simulink model "PID_Tuning"  (R2018a)
settings: Solver=ode45  StartTime=0.0  StopTime=30  RelTol=1e-3  EnableMultiTasking=on
PostLoadFcn:
  | plot_timeseries(Simulation_results);
undefined symbols (not defined in the file or in its folder): A, B, C, D, h, sigbuilder_block
libraries: simulink x4
settings Model: Creator=rbabuska  LastModifiedBy=TU Delf SID
settings DataIOCC: LimitDataPoints=on  SaveFormat=Array
settings OptimizationCC: ExpressionDepthLimit=2147483647  LifeSpan=inf
settings DebuggingCC: AllowSymbolicDim=off  StateNameClashWarn=warning  SFUnexpectedBacktrackingDiag=warning  SFNoUnconditionalDefaultTransitionDiag=warning  SFExecutionAtInitializationDiag=none
settings HardwareCC: ProdBitPerPointer=32  ProdBitPerSizeT=32  ProdBitPerPtrDiffT=32  ProdLargestAtomicFloat=None  ProdIntDivRoundTo=Undefined  ProdEndianess=Unspecified  ProdWordSize=32  ProdHWDeviceType=32-bit Generic
settings ModelReferenceCC: PropagateSignalLabelsOutOfModel=off
settings CodeAppCC: StateflowObjectComments=on
settings GRTTargetCC: TargetLangStandard=C89/C90 (ANSI)  GeneratePreprocessorConditionals=Disable all  CombineOutputUpdateFcns=off  GRTInterface=on
settings ConfigComp: CovMetricSettings=dw  CovHtmlReporting=on  CovSaveCumulativeToWorkspaceVar=on  CovSaveSingleToWorkspaceVar=on  CovExternalEMLEnable=off

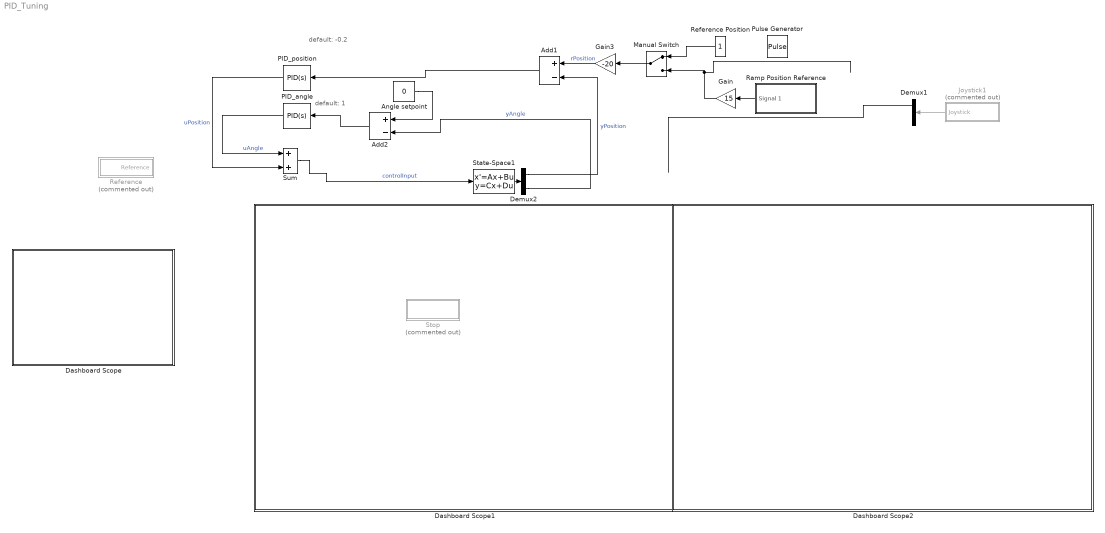
== system PID_Tuning ==
  note: default: -0.2
  note: default: 1
  Add1 : Sum  Inputs=+-
  Add2 : Sum  Inputs=+-
  "Angle setpoint " : Constant  Value=0
  Dashboard Scope : Subsystem  DialogController=hmiCreateDDGDialog  IsWebBlock=on  mask(MWDashboardBlock){webBlockId=8f12994a-5c68-4e4f-80e2-1b29de83f4a9, webBlockType=sdiscope, ShowInitialText=on, HMISrcModelName=PID_Tuning}
      mask prompts: webBlockId "WebBlock Id"; webBlockType "WebBlock Type"; HMISrcModelName "Source Model"
      mask help: SimulinkHMI:dialogs:HMIScopeDialogDesc
      mask Help: helpview([docroot '/mapfiles/simulink.map'], 'hmi_scope')
      mask Display:
      | if strcmp(get_param(bdroot(gcb),'BlockDiagramType'), 'library')
      |     image([(matlabroot) '/toolbox/simulink/hmi/icons/DashboardScope.png']);
      | end
  Dashboard Scope1 : Subsystem  DialogController=hmiCreateDDGDialog  IsWebBlock=on  mask(MWDashboardBlock){webBlockId=26260313-c547-41b7-b078-74ae54bbf42b, webBlockType=sdiscope, ShowInitialText=on, HMISrcModelName=PID_Tuning}
      mask prompts: webBlockId "WebBlock Id"; webBlockType "WebBlock Type"; HMISrcModelName "Source Model"
      mask help: SimulinkHMI:dialogs:HMIScopeDialogDesc
      mask Help: helpview([docroot '/mapfiles/simulink.map'], 'hmi_scope')
      mask Display:
      | if strcmp(get_param(bdroot(gcb),'BlockDiagramType'), 'library')
      |     image([(matlabroot) '/toolbox/simulink/hmi/icons/DashboardScope.png']);
      | end
  Dashboard Scope2 : Subsystem  DialogController=hmiCreateDDGDialog  IsWebBlock=on  mask(MWDashboardBlock){webBlockId=fbac52ec-2b20-4637-bbad-1534b920c4de, webBlockType=sdiscope, ShowInitialText=on, HMISrcModelName=PID_Tuning}
      mask prompts: webBlockId "WebBlock Id"; webBlockType "WebBlock Type"; HMISrcModelName "Source Model"
      mask help: SimulinkHMI:dialogs:HMIScopeDialogDesc
      mask Help: helpview([docroot '/mapfiles/simulink.map'], 'hmi_scope')
      mask Display:
      | if strcmp(get_param(bdroot(gcb),'BlockDiagramType'), 'library')
      |     image([(matlabroot) '/toolbox/simulink/hmi/icons/DashboardScope.png']);
      | end
  Demux1 : Demux  Outputs=2
  Demux2 : Demux  Outputs=2
  Gain : Gain  Gain=15
  Gain3 : Gain  Gain=-20
  Joystick1 : Subsystem  Commented=on
      mask Display: disp('Joystick')
  Manual Switch : ManualSwitch
  PID_angle : simulink/Continuous/PID Controller  Controller=PID  TimeDomain=Continuous-time  SampleTime=-1  IntegratorMethod=Forward Euler  FilterMethod=Forward Euler  Form=Parallel  UseFilter=on  ControllerParametersSource=internal  P=1  I=0  D=1  N=1  InitialConditionSource=internal  InitialConditionForIntegrator=0  InitialConditionForFilter=0  ExternalReset=none  LimitOutput=off  UpperSaturationLimit=inf  LowerSaturationLimit=-inf  LinearizeAsGain=on  AntiWindupMode=none  Kb=1  TrackingMode=off  Kt=1  PParamMin=[]  PParamMax=[]  IParamMin=[]  IParamMax=[]  DParamMin=[]  DParamMax=[]  NParamMin=[]  NParamMax=[]  KbParamMin=[]  KbParamMax=[]  KtParamMin=[]  KtParamMax=[]  POutMin=[]  POutMax=[]  IOutMin=[]  IOutMax=[]  DOutMin=[]  DOutMax=[]  NOutMin=[]  NOutMax=[]  KbOutMin=[]  KbOutMax=[]  KtOutMin=[]  KtOutMax=[]  IntegratorOutMin=[]  IntegratorOutMax=[]  FilterOutMin=[]  FilterOutMax=[]  SumOutMin=[]  SumOutMax=[]  SumI1OutMin=[]  SumI1OutMax=[]  SumI2OutMin=[]  SumI2OutMax=[]  SumI3OutMin=[]  SumI3OutMax=[]  SumDOutMin=[]  SumDOutMax=[]  SaturationOutMin=[]  SaturationOutMax=[]  IntegratorContinuousStateAttributes=''  IntegratorStateMustResolveToSignalObject=off  IntegratorRTWStateStorageClass=Auto  FilterContinuousStateAttributes=''  FilterStateMustResolveToSignalObject=off  FilterRTWStateStorageClass=Auto  DifferentiatorICPrevScaledInput=0  DifferentiatorOutMin=[]  DifferentiatorOutMax=[]  FilterDiffOutCoefMin=[]  FilterDiffOutCoefMax=[]  SumDenOutMin=[]  SumDenOutMax=[]  SumNumOutMin=[]  SumNumOutMax=[]  ReciprocalOutMin=[]  ReciprocalOutMax=[]  DivideOutMin=[]  DivideOutMax=[]  TunerSelectOption=Transfer Function Based (PID Tuner App)
  PID_position : simulink/Continuous/PID Controller  Controller=PID  TimeDomain=Continuous-time  SampleTime=-1  IntegratorMethod=Forward Euler  FilterMethod=Forward Euler  Form=Parallel  UseFilter=on  ControllerParametersSource=internal  P=-0.2  I=0  D=0  N=1  InitialConditionSource=internal  InitialConditionForIntegrator=0  InitialConditionForFilter=0  ExternalReset=none  LimitOutput=off  UpperSaturationLimit=inf  LowerSaturationLimit=-inf  LinearizeAsGain=on  AntiWindupMode=none  Kb=1  TrackingMode=off  Kt=1  PParamMin=[]  PParamMax=[]  IParamMin=[]  IParamMax=[]  DParamMin=[]  DParamMax=[]  NParamMin=[]  NParamMax=[]  KbParamMin=[]  KbParamMax=[]  KtParamMin=[]  KtParamMax=[]  POutMin=[]  POutMax=[]  IOutMin=[]  IOutMax=[]  DOutMin=[]  DOutMax=[]  NOutMin=[]  NOutMax=[]  KbOutMin=[]  KbOutMax=[]  KtOutMin=[]  KtOutMax=[]  IntegratorOutMin=[]  IntegratorOutMax=[]  FilterOutMin=[]  FilterOutMax=[]  SumOutMin=[]  SumOutMax=[]  SumI1OutMin=[]  SumI1OutMax=[]  SumI2OutMin=[]  SumI2OutMax=[]  SumI3OutMin=[]  SumI3OutMax=[]  SumDOutMin=[]  SumDOutMax=[]  SaturationOutMin=[]  SaturationOutMax=[]  IntegratorContinuousStateAttributes=''  IntegratorStateMustResolveToSignalObject=off  IntegratorRTWStateStorageClass=Auto  FilterContinuousStateAttributes=''  FilterStateMustResolveToSignalObject=off  FilterRTWStateStorageClass=Auto  DifferentiatorICPrevScaledInput=0  DifferentiatorOutMin=[]  DifferentiatorOutMax=[]  FilterDiffOutCoefMin=[]  FilterDiffOutCoefMax=[]  SumDenOutMin=[]  SumDenOutMax=[]  SumNumOutMin=[]  SumNumOutMax=[]  ReciprocalOutMin=[]  ReciprocalOutMax=[]  DivideOutMin=[]  DivideOutMax=[]  TunerSelectOption=Transfer Function Based (PID Tuner App)
  Pulse Generator : DiscretePulseGenerator  PulseType=Time based  Amplitude=15  Period=30  PulseWidth=50  PhaseDelay=2
  Ramp Position Reference : Subsystem  Tag=STV Subsys  LoadFcn=sigbuilder_block('load');  StartFcn=sigbuilder_block('start');  StopFcn=sigbuilder_block('stop');  ClipboardFcn=sigbuilder_block('clipboard');  mask(Sigbuilder block){tuvar=[0:10]}
      mask help: Simulink:masks:SigbuilderBlock_MD
      mask init:
      | if ~strcmp(get_param(bdroot(gcbh),'SimulationStatus'),'stopped') tuvar = sigbuilder_block('maskInit'); end
      settings: CopyFcn=sigbuilder_block('copy');  DeleteFcn=sigbuilder_block('delete');  ModelCloseFcn=sigbuilder_block('modelClose');  PreSaveFcn=sigbuilder_block('preSave');  PauseFcn=sigbuilder_block('pause');  ContinueFcn=sigbuilder_block('continue');  NameChangeFcn=sigbuilder_block('namechange');  OpenFcn=sigbuilder_block('open',[718.5 180 550.5 399.75 ]);  CloseFcn=sigbuilder_block('close');
      mask Display: plot(0, 0, 100, 100,[2, 2, 32, 32, 2], [68, 8, 8, 68, 68],[32, 2], [38, 38], [32, 19, 2],[53, 60, 44], [32, 17, 17, 2],[16, 16, 31, 31]);txt = getActiveGroup(gcbh);text(2, 100, txt,'verticalAlignment', 'top');
  Reference : Subsystem  Commented=on
      mask Display: disp('Reference')
  Reference Position : Constant
  State-Space1 : StateSpace  A=A  B=B  C=C  D=D  InitialCondition=0
  Stop : Subsystem  Commented=on
      mask Display: disp('Stop')
  Sum : Sum
  wires:
  Demux2/2 -> Add2/2  "yAngle"
  Demux2/1 -> Add1/2  "yPosition"
  Sum/1 -> State-Space1/1  "controlInput"
  "Angle setpoint "/1 -> Add2/1
  PID_position/1 -> Sum/2  "uPosition"
  PID_angle/1 -> Sum/1  "uAngle"
  Gain3/1 -> Add1/1  "rPosition"
  Reference Position/1 -> Manual Switch/1
  Gain/1 -> Manual Switch/2
  Add2/1 -> PID_angle/1
  Ramp Position Reference/1(Signal 1) -> Gain/1
  Add1/1 -> PID_position/1
  Joystick1/1(Joystick) -> Demux1/1
  Demux1/1 -> ?
  State-Space1/1 -> Demux2/1
  Manual Switch/1 -> Gain3/1

== system PID_Tuning/Dashboard Scope ==

== system PID_Tuning/Dashboard Scope1 ==

== system PID_Tuning/Dashboard Scope2 ==

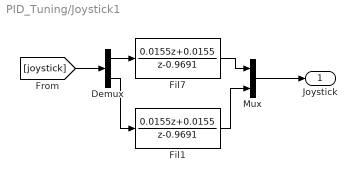
== system PID_Tuning/Joystick1 ==
  Demux : Demux  Outputs=2
  Fil1 : DiscreteTransferFcn  Numerator=[0.0155 0.0155]  Denominator=[1 -0.9691]  SampleTime=h
  Fil7 : DiscreteTransferFcn  Numerator=[0.0155 0.0155]  Denominator=[1 -0.9691]  SampleTime=h
  Mux : Mux  Inputs=2
  Joystick : Outport
  wires:
  Mux/1 -> Joystick/1
  Fil1/1 -> Mux/2
  Demux/2 -> Fil1/1
  Demux/1 -> Fil7/1
  [joystick] -> Demux/1
  Fil7/1 -> Mux/1

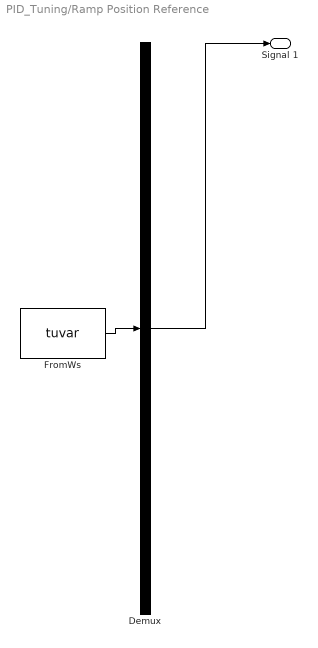
== system PID_Tuning/Ramp Position Reference ==
  Demux : Demux  Tag=STV Demux  Outputs=1
  FromWs : FromWorkspace  Tag=STV FromWs  VariableName=tuvar  SampleTime=0
      SigBuilderData=|
      | common.afterFinalStr = 'Extrapolate'
      | common.sampleTime = 0
      | dataSet.timeRange = [0 30]
      | dataSet.name = 'Group 1'
      | sbobj.Groups.Name = 'Group 1'
      | sbobj.Groups.Signals.Name = 'Signal 1'
      | sbobj.Groups.Signals.XData = [0 2 3.5 10 30]
      | sbobj.Groups.Signals.YData = [0 0 1 1 1.005]
      | sbobj.Groups.TimeRange = [0 30]
  Signal 1 : Outport  Tag=STV Outport
  wires:
  Demux/1 -> Signal 1/1
  FromWs/1 -> Demux/1

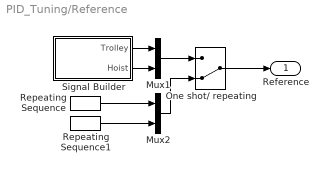
== system PID_Tuning/Reference ==
  Mux1 : Mux  Inputs=2
  Mux2 : Mux  Inputs=2
  One shot/ repeating : ManualSwitch  CurrentSetting=0
  Repeating Sequence : simulink/Sources/Repeating Sequence  rep_seq_t="[0    4.5000   12.5000   22.5000   30.5000   36.0000]"  rep_seq_y="[0         0    1.5000    1.5000         0         0]"
  Repeating Sequence1 : simulink/Sources/Repeating Sequence  rep_seq_t="[0     2     7    10    15    20    25    28    33    36]"  rep_seq_y="[0         0   -0.8000   -0.8000    0.3400    0.3400   -0.8000  -0.8000         0         0]"
  Signal Builder : Subsystem  Tag=STV Subsys  LoadFcn=sigbuilder_block('load');  StartFcn=sigbuilder_block('start');  StopFcn=sigbuilder_block('stop');  ClipboardFcn=sigbuilder_block('clipboard');  mask(Sigbuilder block){tuvar=[0:10]}
      mask help: Sigbuilder GUI
      mask init:
      | if ~strcmp(get_param(bdroot(gcb),'SimulationStatus'),'stopped') tuvar = sigbuilder_block('maskInit'); end
      settings: CopyFcn=sigbuilder_block('copy');  DeleteFcn=sigbuilder_block('delete');  ModelCloseFcn=sigbuilder_block('modelClose');  PreSaveFcn=sigbuilder_block('preSave');  PauseFcn=sigbuilder_block('pause')  ContinueFcn=sigbuilder_block('continue')  NameChangeFcn=sigbuilder_block('namechange');  OpenFcn=sigbuilder_block('open',[50.25 82.5 519.75 399.75 ]);  CloseFcn=sigbuilder_block('close');
      mask Display: plot(0, 0, 100, 100,[2, 2, 32, 32, 2], [68, 8, 8, 68, 68],[32, 2], [38, 38], [32, 19, 2],[53, 60, 44], [32, 17, 17, 2],[16, 16, 31, 31]);txt = getActiveGroup(gcbh);text(2, 100, txt,'verticalAlignment', 'top');
  Reference : Outport
  wires:
  Repeating Sequence1/1 -> Mux2/2
  Mux2/1 -> One shot/ repeating/2
  Repeating Sequence/1 -> Mux2/1
  Mux1/1 -> One shot/ repeating/1
  One shot/ repeating/1 -> Reference/1
  Signal Builder/1(Trolley) -> Mux1/1
  Signal Builder/2(Hoist) -> Mux1/2

== system PID_Tuning/Stop ==

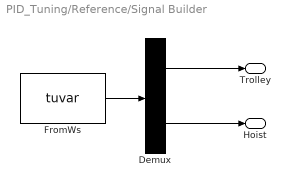
== system PID_Tuning/Reference/Signal Builder ==
  Demux : Demux  Tag=STV Demux  Outputs=2
  FromWs : FromWorkspace  Tag=STV FromWs  VariableName=tuvar  SampleTime=0
      SigBuilderData=|
      | dataSet.timeRange = [0 36]
      | dataSet.name = 'Group 1'
      | sbobj.Groups.Name = 'Group 1'
      | sbobj.Groups.Signals(1).Name = 'Trolley'
      | sbobj.Groups.Signals(1).XData = [0 4.5 12.5 22.5 30.5 36]
      | sbobj.Groups.Signals(1).YData = [0 0 1.5 1.5 0 0]
      | sbobj.Groups.Signals(2).Name = 'Hoist'
      | sbobj.Groups.Signals(2).XData = [0 2 7 10 15 20 25 28 33 36]
      | sbobj.Groups.Signals(2).YData = [0 0 -0.8 -0.8 0.34 0.34 -0.8 -0.8 0 0]
  Trolley : Outport  Tag=STV Outport
  Hoist : Outport  Tag=STV Outport  Port=2
  wires:
  Demux/2 -> Hoist/1
  Demux/1 -> Trolley/1
  FromWs/1 -> Demux/1
